simulink model "lv_test"  (R2019b)
settings: Solver=ode4  StartTime=0.0  StopTime=1  FixedStep=Tn  RelTol=1e-3
settings Model: Creator=a4327  LastModifiedBy=a4327

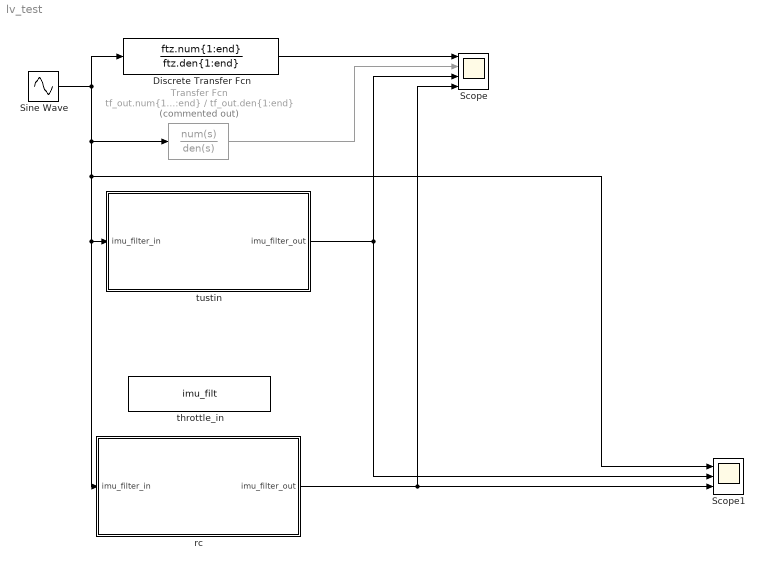
== system lv_test ==
  Discrete Transfer Fcn : DiscreteTransferFcn  Numerator=ftz.num{1:end}  Denominator=ftz.den{1:end}
  Scope : Scope  NumInputPorts=4
  Scope1 : Scope  NumInputPorts=3
  Sine Wave : Sin  Frequency=2*pi*40  SampleTime=0
  Transfer Fcn : TransferFcn  Commented=on  Numerator=tf_out.num{1:end}  Denominator=tf_out.den{1:end}
  rc : MATLAB Function  TreatAsAtomicUnit=on
  throttle_in : DataStoreMemory  DataStoreName=imu_filt  ReadBeforeWriteMsg=warning  WriteAfterWriteMsg=warning  WriteAfterReadMsg=warning  InitialValue=imu_filt  VectorParams1D=off  ShowAdditionalParam=off  OutDataTypeStr=double
  tustin : MATLAB Function  TreatAsAtomicUnit=on
  wires:
  Discrete Transfer Fcn/1 -> Scope/1
  Transfer Fcn/1 -> Scope/2
  Sine Wave/1 -> Scope1/1, rc/1(imu_filter_in), tustin/1(imu_filter_in), Transfer Fcn/1, Discrete Transfer Fcn/1
  tustin/1(imu_filter_out) -> Scope1/2, Scope/3
  rc/1(imu_filter_out) -> Scope/4, Scope1/3

== matlab function lv_test/tustin ==
  data: imu_filter_in input; imu_filter_out output
function imu_filter_out = imu_filter(imu_filter_in)
% ftz.num{1:end}
% ftz.den{1:end}
% persistent
persistent imu_filter_in_buff
persistent imu_filter_out_buff
    if isempty(imu_filter_in_buff)
        imu_filter_in_buff = zeros(3,1);
    end
    if isempty(imu_filter_out_buff)
        imu_filter_out_buff = zeros(3,1);
    end 
    
    

imu_filter_in_buff(1,:)=imu_filter_in_buff(2,:);
imu_filter_in_buff(2,:)=imu_filter_in_buff(3,:);
imu_filter_in_buff(3,:)=imu_filter_in;
imu_filter_out_buff(1,:)=imu_filter_out_buff(2,:);
imu_filter_out_buff(2,:)=imu_filter_out_buff(3,:);
imu_filter_out=imu_filter_in_buff(3,:)*0.1287+imu_filter_in_buff(2,:)*0.2574+imu_filter_in_buff(1,:)*0.1287-imu_filter_out_buff(2,:)*- 0.7613-imu_filter_out_buff(1,:)*0.276;
% imu_filter_out=imu_filter_in_buff(3,:)*0.008771+imu_filter_in_buff(2,:)*0.01754+imu_filter_in_buff(1,:)*0.008771-imu_filter_out_buff(2,:)*- 1.718-imu_filter_out_buff(1,:)*0.7533;

imu_filter_out_buff(3,:)=imu_filter_out;

== matlab function lv_test/rc ==
  data: imu_filter_in input; imu_filter_out output; imu_filt data_store_memory
function imu_filter_out = imu_filter(imu_filter_in)
% ftz.num{1:end}
% ftz.den{1:end}
% persistent
persistent imu_filter_temp
persistent dt
global imu_filt
    if isempty(imu_filter_temp)
        imu_filter_temp = zeros(1,1);
    end
    
   if isempty(dt)
        dt = 0.004;
    end

  rc=1/(2*pi*imu_filt);
  alpha=dt/(dt+rc);
  imu_filter_temp=imu_filter_temp+(imu_filter_in-imu_filter_temp)*alpha;
  imu_filter_out=imu_filter_temp;  
    
%     
% 
% imu_filter_in_buff(1,:)=imu_filter_in_buff(2,:);
% imu_filter_in_buff(2,:)=imu_filter_in_buff(3,:);
% imu_filter_in_buff(3,:)=imu_filter_in;
% imu_filter_out_buff(1,:)=imu_filter_out_buff(2,:);
% imu_filter_out_buff(2,:)=imu_filter_out_buff(3,:);
% % imu_filter_out=imu_filter_in_buff(3,:)*0.1287+imu_filter_in_buff(2,:)*0.2574+imu_filter_in_buff(1,:)*0.1287-imu_filter_out_buff(2,:)*- 0.7613-imu_filter_out_buff(1,:)*0.276;
% imu_filter_out=imu_filter_in_buff(3,:)*0.008771+imu_filter_in_buff(2,:)*0.01754+imu_filter_in_buff(1,:)*0.008771-imu_filter_out_buff(2,:)*- 1.718-imu_filter_out_buff(1,:)*0.7533;
% % imu_filter_out=imu_filter_in_buff(3,:)*0.003613+imu_filter_in_buff(2,:)*0.007225+imu_filter_in_buff(1,:)*0.003613-imu_filter_out_buff(2,:)*- 1.823-imu_filter_out_buff(1,:)*0.8374;
% 
% imu_filter_out_buff(3,:)=imu_filter_out;
